simulink model "SimuModel_E_compuTorqForward"  (Simulink 9.3)
settings: Solver=ode23  StartTime=0.0  StopTime=t_d  MaxStep=Tc  RelTol=1e-8  AbsTol=1e-8
values from neighbouring files (symbols this model uses):
  F_e = K_r*k_t*inv(R_a)*k_v*K_r    [InitVariable_E.m]
  F_v = K_r*diag([0.01 0.01])*K_r    [InitVariable_E.m]
  g = 9.81    [InitVariable_E.m]
  G_r = K_r*k_t*inv(R_a)*G_v    [InitVariable_E.m]
  k_fa = K_r*k_v*inv(K_v)    [InitVariable_E.m]
  k_fp = k_tp    [InitVariable_E.m]
  k_fv = k_tv    [InitVariable_E.m]
  K_p = 5*diag([1 1])    [InitVariable_E.m]
  K_pr = R_a*inv(k_t*K_r)    [InitVariable_E.m]
  k_tp = K_r*k_tp    [InitVariable_E.m]
  k_tv = K_r*k_tv    [InitVariable_E.m]
  K_v = 10*diag([1 1])    [InitVariable_E.m]
  q_i = [-1.4706; 2.9413]    [InitVariable_E.m]
  Tc = 0.001    [InitVariable_E.m]
  Ts = Tc    (= 0.001)    [InitVariable_E.m]
undefined symbols (not defined in the file or in its folder): a, Ad, Bd, BMatrix, Cd, Dd, pi_l, pi_m
settings Model: Creator=luigivillani  LastModifiedBy=yuzg  ExtModeAutoUpdateStatusClock=off
settings SolverCC: AutoScaleAbsTol=off  InitialStep=0.1*Tc
settings DataIOCC: SaveOutput=off  SaveTime=off
settings OptimizationCC: BlockReduction=off  BooleanDataType=off  ExpressionDepthLimit=2147483647  InitFltsAndDblsToZero=on
settings DebuggingCC: SaveWithParameterizedLinksMsg=none  SignalResolutionControl=TryResolveAllWithWarning  MultiTaskDSMMsg=warning  MultiTaskCondExecSysMsg=none  StateNameClashWarn=warning
settings HardwareCC: TargetUnknown=on
settings SFSimCC: SimUseLocalCustomCode=on
settings RTWCC: RTWUseLocalCustomCode=on
settings GRTTargetCC: TargetFcnLib=ansi_tfl_tmw.mat
settings ConfigComp: CovExternalEMLEnable=on

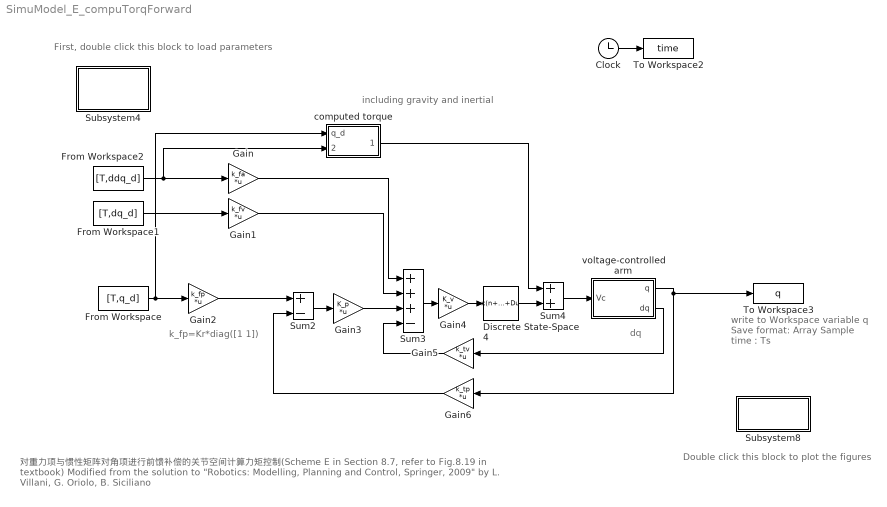
== system SimuModel_E_compuTorqForward ==
  note: including gravity and inertial
  note: k_fp=Kr*diag([1 1])
  note: Double click this block to plot the figures
  note: First, double click this block to load parameters
  note: write to Workspace variable q
      | Save format: Array
      | Sample time：Ts
  note: dq
  note: 对重力项与惯性矩阵对角项进行前馈补偿的关节空间计算力矩控制(Scheme E in Section 8.7, refer to Fig.8.19 in textbook)
      | Modified from the solution to "Robotics: Modelling, Planning and Control, Springer, 2009" by L. Villani, G. Oriolo, B. Siciliano
  Clock : Clock
  Discrete State-Space4 : DiscreteStateSpace  A=Ad  B=Bd  C=Cd  D=Dd  InitialCondition=[0 0]  SampleTime=Tc
      mask Display: disp('PI')
  From Workspace : FromWorkspace  VariableName=[T,q_d]  SampleTime=Tc
  From Workspace1 : FromWorkspace  VariableName=[T,dq_d]  SampleTime=Tc
  From Workspace2 : FromWorkspace  VariableName=[T,ddq_d]  SampleTime=Tc
  Gain : Gain  Gain=k_fa  Multiplication=Matrix(K*u)  SampleTime=Tc
      mask Display: disp('k_fa')
  Gain1 : Gain  Gain=k_fv  Multiplication=Matrix(K*u)  SampleTime=Tc
      mask Display: disp('k_fv')
  Gain2 : Gain  Gain=k_fp  Multiplication=Matrix(K*u)  SampleTime=Tc
      mask Display: disp('k_fp')
  Gain3 : Gain  Gain=K_p  Multiplication=Matrix(K*u)  SampleTime=Tc
      mask Display: disp('K_p')
  Gain4 : Gain  Gain=K_v  Multiplication=Matrix(K*u)  SampleTime=Tc
      mask Display: disp('K_v')
  Gain5 : Gain  Gain=k_tv  Multiplication=Matrix(K*u)  SampleTime=Tc
      mask Display: disp('k_tv')
  Gain6 : Gain  Gain=k_tp  Multiplication=Matrix(K*u)  SampleTime=Tc
      mask Display: disp('k_tp')
  Subsystem4 : Subsystem
      settings: OpenFcn=clear all;c=0;InitVariable;
      mask Display: disp('K_p = 5\nK_v = 10')
  Subsystem8 : Subsystem
      settings: OpenFcn=PlotFigure;
      mask Display: disp('plot')
  Sum2 : Sum  Inputs=+-  SaturateOnIntegerOverflow=on  InputSameDT=on  OutDataTypeStr=Inherit: Same as first input
  Sum3 : Sum  Inputs=+++-  SaturateOnIntegerOverflow=on  InputSameDT=on  OutDataTypeStr=Inherit: Same as first input
  Sum4 : Sum  SaturateOnIntegerOverflow=on  InputSameDT=on  OutDataTypeStr=Inherit: Same as first input
  To Workspace2 : ToWorkspace  VariableName=time  SampleTime=Ts
      settings: MaxDataPoints=5001
  To Workspace3 : ToWorkspace  VariableName=q  SampleTime=Ts
      settings: MaxDataPoints=5001
  computed torque : Subsystem
      mask Display: disp('tau_d')
  voltage-controlled arm : Subsystem
      mask Display: disp('Manipulator')
  wires:
  Sum2/1 -> Gain3/1
  Clock/1 -> To Workspace2/1
  Gain6/1 -> Sum2/2
  voltage-controlled arm/2(dq) -> Gain5/1
  Gain4/1 -> Discrete State-Space4/1
  voltage-controlled arm/1(q) -> To Workspace3/1, Gain6/1
  From Workspace/1 -> computed torque/1(q_d), Gain2/1
  Gain2/1 -> Sum2/1
  Gain/1 -> Sum3/1
  Gain1/1 -> Sum3/2
  From Workspace1/1 -> Gain1/1
  From Workspace2/1 -> computed torque/2(ddq_d), Gain/1
  Sum3/1 -> Gain4/1
  Gain5/1 -> Sum3/4
  Gain3/1 -> Sum3/3
  Sum4/1 -> voltage-controlled arm/1(Vc)
  Discrete State-Space4/1 -> Sum4/2
  computed torque/1(tau_d) -> Sum4/1

== system SimuModel_E_compuTorqForward/Subsystem4 ==
  note: start

== system SimuModel_E_compuTorqForward/Subsystem8 ==
  note: start

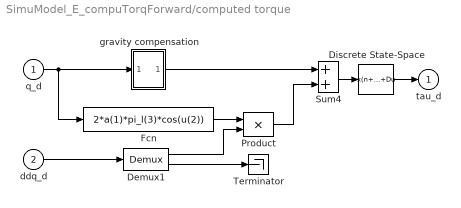
== system SimuModel_E_compuTorqForward/computed torque ==
  q_d : Inport
  ddq_d : Inport  Port=2
  Demux1 : Demux  Outputs=2
  Discrete State-Space : DiscreteStateSpace  A=0  B=zeros(1,2)  C=zeros(2,1)  D=K_pr  SampleTime=Tc
      mask Display: disp('K_pr')
  Fcn : Fcn  Expr=2*a(1)*pi_l(3)*cos(u(2))
  Product : Product  SaturateOnIntegerOverflow=on  RndMeth=Zero  InputSameDT=on  OutDataTypeStr=Inherit: Same as first input
  Sum4 : Sum  SaturateOnIntegerOverflow=on  InputSameDT=on  OutDataTypeStr=Inherit: Same as first input
  Terminator : Terminator
  gravity compensation : Subsystem
      mask Display: disp('g(q)')
  tau_d : Outport  InitialOutput=0
  wires:
  Discrete State-Space/1 -> tau_d/1
  ddq_d/1 -> Demux1/1
  Fcn/1 -> Product/1
  Demux1/1 -> Product/2
  gravity compensation/1(out_1) -> Sum4/1
  Product/1 -> Sum4/2
  Sum4/1 -> Discrete State-Space/1
  q_d/1 -> gravity compensation/1(in_1), Fcn/1
  Demux1/2 -> Terminator/1

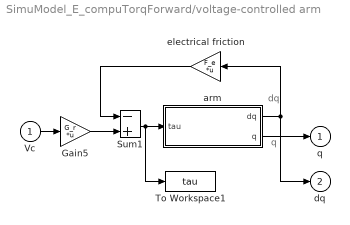
== system SimuModel_E_compuTorqForward/voltage-controlled arm ==
  note: dq
  note: q
  Vc : Inport
  Gain5 : Gain  Gain=G_r  Multiplication=Matrix(K*u)  SampleTime=0
      mask Display: disp('G_r')
  Sum1 : Sum  Inputs=-+  SaturateOnIntegerOverflow=on  InputSameDT=on  OutDataTypeStr=Inherit: Same as first input
  To Workspace1 : ToWorkspace  VariableName=tau  SampleTime=Ts
      settings: MaxDataPoints=5001
  arm : Subsystem
      mask Display: disp('inv(B(q))(tau-tau'')')
  electrical friction : Gain  Gain=F_e  Multiplication=Matrix(K*u)  SampleTime=0
      mask Display: disp('F_e')
  q : Outport  InitialOutput=0
  dq : Outport  Port=2  InitialOutput=0
  wires:
  Vc/1 -> Gain5/1
  Gain5/1 -> Sum1/2
  electrical friction/1 -> Sum1/1
  arm/2("q ") -> q/1
  arm/1(dq) -> dq/1, electrical friction/1
  Sum1/1 -> To Workspace1/1, arm/1(tau)

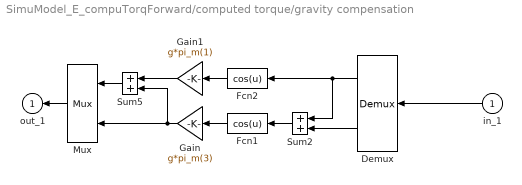
== system SimuModel_E_compuTorqForward/computed torque/gravity compensation ==
  in_1 : Inport
  Demux : Demux  Outputs=2
  Fcn1 : Fcn  Expr=cos(u)
  Fcn2 : Fcn  Expr=cos(u)
  Gain : Gain  Gain=g*pi_m(3)  SaturateOnIntegerOverflow=on  OutDataTypeStr=Inherit: Same as input  ParamDataTypeStr=Inherit: Same as input
      mask Display: disp('k_2')
  Gain1 : Gain  Gain=g*pi_m(1)  SaturateOnIntegerOverflow=on  OutDataTypeStr=Inherit: Same as input  ParamDataTypeStr=Inherit: Same as input
      mask Display: disp('k_1')
  Mux : Mux  Inputs=2
  Sum2 : Sum  SaturateOnIntegerOverflow=on  InputSameDT=on  OutDataTypeStr=Inherit: Same as first input
  Sum5 : Sum  SaturateOnIntegerOverflow=on  InputSameDT=on  OutDataTypeStr=Inherit: Same as first input
  out_1 : Outport  InitialOutput=0
  wires:
  in_1/1 -> Demux/1
  Demux/2 -> Sum2/2
  Sum2/1 -> Fcn1/1
  Fcn1/1 -> Gain/1
  Fcn2/1 -> Gain1/1
  Demux/1 -> Fcn2/1, Sum2/1
  Gain1/1 -> Sum5/1
  Sum5/1 -> Mux/1
  Gain/1 -> Mux/2, Sum5/2
  Mux/1 -> out_1/1

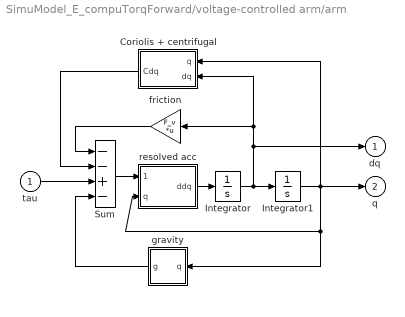
== system SimuModel_E_compuTorqForward/voltage-controlled arm/arm ==
  tau : Inport
  Coriolis + centrifugal : Subsystem
      mask Display: disp('C(q,dq)dq')
  Integrator : Integrator  InitialCondition=[0 0]  ZeroCross=off
  Integrator1 : Integrator  InitialCondition=q_i  ZeroCross=off
  Sum : Sum  Inputs=--+-  SaturateOnIntegerOverflow=on  InputSameDT=on  OutDataTypeStr=Inherit: Same as first input
  friction : Gain  Gain=F_v  Multiplication=Matrix(K*u)  SaturateOnIntegerOverflow=on  OutDataTypeStr=Inherit: Same as input  ParamDataTypeStr=Inherit: Same as input
      mask Display: disp('F_v')
  gravity : Subsystem
      mask Display: disp('g(q)')
  resolved acc : Subsystem
      mask Display: disp('inv(B(q))')
  dq : Outport  InitialOutput=0
  "q " : Outport  Port=2  InitialOutput=0
  wires:
  Coriolis + centrifugal/1(Cdq) -> Sum/2
  tau/1 -> Sum/3
  Integrator1/1 -> Coriolis + centrifugal/1(q), resolved acc/2(q), gravity/1(q), "q "/1
  resolved acc/1(ddq) -> Integrator/1
  Integrator/1 -> Integrator1/1, dq/1, Coriolis + centrifugal/2(dq), friction/1
  Sum/1 -> resolved acc/1(tau-tau')
  friction/1 -> Sum/1
  gravity/1(g) -> Sum/4

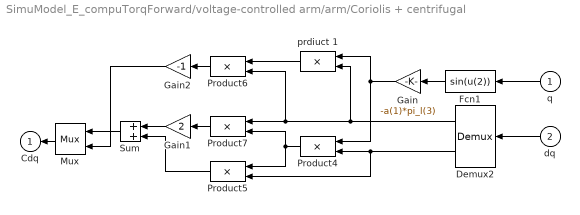
== system SimuModel_E_compuTorqForward/voltage-controlled arm/arm/Coriolis + centrifugal ==
  q : Inport
  dq : Inport  Port=2
  Demux2 : Demux  Outputs=2
  Fcn1 : Fcn  Expr=sin(u(2))
  Gain : Gain  Gain=-a(1)*pi_l(3)  SaturateOnIntegerOverflow=on  OutDataTypeStr=Inherit: Same as input  ParamDataTypeStr=Inherit: Same as input
      mask Display: disp('k_3')
  Gain1 : Gain  Gain=2  SaturateOnIntegerOverflow=on  OutDataTypeStr=Inherit: Same as input  ParamDataTypeStr=Inherit: Same as input
  Gain2 : Gain  Gain=-1  SaturateOnIntegerOverflow=on  OutDataTypeStr=Inherit: Same as input  ParamDataTypeStr=Inherit: Same as input
  Mux : Mux  Inputs=2
  Product{4..7} (4 alike) : Product  SaturateOnIntegerOverflow=on  RndMeth=Zero  InputSameDT=on  OutDataTypeStr=Inherit: Same as first input
  Sum : Sum  SaturateOnIntegerOverflow=on  InputSameDT=on  OutDataTypeStr=Inherit: Same as first input
  prdiuct 1 : Product  SaturateOnIntegerOverflow=on  RndMeth=Zero  InputSameDT=on  OutDataTypeStr=Inherit: Same as first input
  Cdq : Outport  InitialOutput=0
  wires:
  dq/1 -> Demux2/1
  Gain2/1 -> Mux/2
  Product6/1 -> Gain2/1
  Mux/1 -> Cdq/1
  Sum/1 -> Mux/1
  Product5/1 -> Sum/2
  Gain1/1 -> Sum/1
  Product7/1 -> Gain1/1
  Demux2/1 -> prdiuct 1/2, Product6/2, Product7/1
  Demux2/2 -> Product4/2, Product5/2
  prdiuct 1/1 -> Product6/1
  Gain/1 -> prdiuct 1/1, Product4/1
  Fcn1/1 -> Gain/1
  q/1 -> Fcn1/1
  Product4/1 -> Product5/1, Product7/2

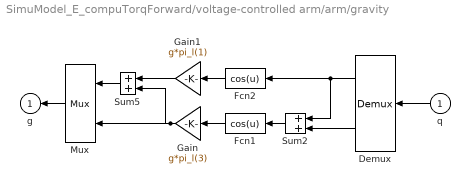
== system SimuModel_E_compuTorqForward/voltage-controlled arm/arm/gravity ==
  q : Inport
  Demux : Demux  Outputs=2
  Fcn1 : Fcn  Expr=cos(u)
  Fcn2 : Fcn  Expr=cos(u)
  Gain : Gain  Gain=g*pi_l(3)  SaturateOnIntegerOverflow=on  OutDataTypeStr=Inherit: Same as input  ParamDataTypeStr=Inherit: Same as input
      mask Display: disp('k_2')
  Gain1 : Gain  Gain=g*pi_l(1)  SaturateOnIntegerOverflow=on  OutDataTypeStr=Inherit: Same as input  ParamDataTypeStr=Inherit: Same as input
      mask Display: disp('k_1')
  Mux : Mux  Inputs=2
  Sum2 : Sum  SaturateOnIntegerOverflow=on  InputSameDT=on  OutDataTypeStr=Inherit: Same as first input
  Sum5 : Sum  SaturateOnIntegerOverflow=on  InputSameDT=on  OutDataTypeStr=Inherit: Same as first input
  g : Outport  InitialOutput=0
  wires:
  q/1 -> Demux/1
  Demux/2 -> Sum2/2
  Sum2/1 -> Fcn1/1
  Fcn1/1 -> Gain/1
  Fcn2/1 -> Gain1/1
  Demux/1 -> Fcn2/1, Sum2/1
  Gain1/1 -> Sum5/1
  Sum5/1 -> Mux/1
  Gain/1 -> Sum5/2, Mux/2
  Mux/1 -> g/1

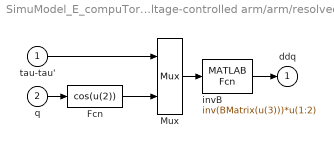
== system SimuModel_E_compuTorqForward/voltage-controlled arm/arm/resolved acc ==
  tau-tau' : Inport
  q : Inport  Port=2
  Fcn : Fcn  Expr=cos(u(2))
  Mux : Mux  Inputs=[2,1]
  "invB " : MATLABFcn  MATLABFcn=inv(BMatrix(u(3)))*u(1:2)  OutputDimensions=2
      mask Display: disp('inv(B(q))')
  ddq : Outport  InitialOutput=0
  wires:
  Fcn/1 -> Mux/2
  q/1 -> Fcn/1
  "invB "/1 -> ddq/1
  tau-tau'/1 -> Mux/1
  Mux/1 -> "invB "/1
